simulink model "TP_1"  (R2018a)
settings: Solver=VariableStepAuto  StartTime=0.0  StopTime=500  RelTol=1e-3
settings Model: Creator=akumar2017  LastModifiedBy=Frank NGO

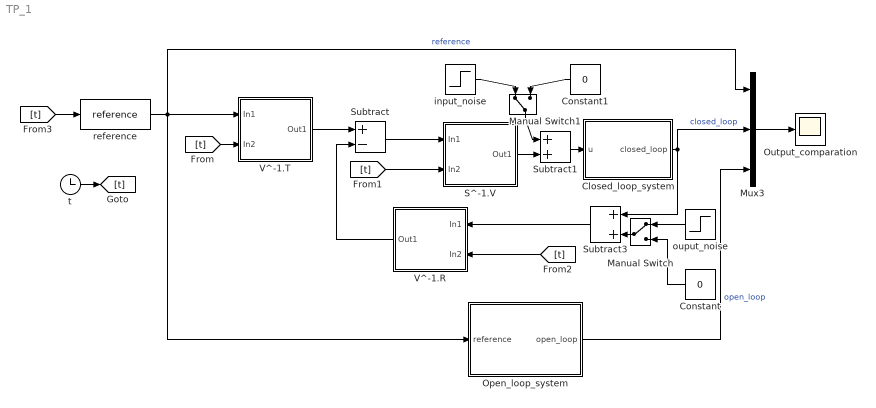
== system TP_1 ==
  Closed_loop_system : Subsystem
  Constant : Constant  Value=0
  Constant1 : Constant  Value=0
  Manual Switch : ManualSwitch
  Manual Switch1 : ManualSwitch
  Mux3 : Mux  Inputs=3
  Open_loop_system : Subsystem
  Output_comparation : Scope
  S^-1.V : Subsystem
  Subtract : Sum  Inputs=+-
  Subtract1 : Sum
  Subtract3 : Sum
  V^-1.R : Subsystem
  V^-1.T : Subsystem
  input_noise : Step  Time=100  After=5  SampleTime=0
  ouput_noise : Step  Time=200  After=0.09  SampleTime=0
  reference : MATLABFcn  MATLABFcn=reference  OutputDimensions=1
  t : Clock
  wires:
  Closed_loop_system/1(closed_loop) -> Subtract3/1, Mux3/2  "closed_loop"
  [t] -> V^-1.T/2(In2)
  [t] -> S^-1.V/2(In2)
  t/1 -> [t]
  [t] -> V^-1.R/2(In2)
  V^-1.T/1(Out1) -> Subtract/1
  V^-1.R/1(Out1) -> Subtract/2
  Subtract/1 -> S^-1.V/1(In1)
  Mux3/1 -> Output_comparation/1
  [t] -> reference/1
  S^-1.V/1(Out1) -> Subtract1/2
  Subtract1/1 -> Closed_loop_system/1(u)
  input_noise/1 -> Manual Switch1/1
  reference/1 -> Open_loop_system/1(reference), Mux3/1, V^-1.T/1(In1)  "reference"
  Subtract3/1 -> V^-1.R/1(In1)
  ouput_noise/1 -> Manual Switch/1
  Open_loop_system/1(open_loop) -> Mux3/3  "open_loop"
  Constant/1 -> Manual Switch/2
  Manual Switch/1 -> Subtract3/2
  Manual Switch1/1 -> Subtract1/1
  Constant1/1 -> Manual Switch1/2

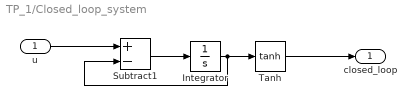
== system TP_1/Closed_loop_system ==
  u : Inport
  Integrator : Integrator
  Subtract1 : Sum  Inputs=+-
  Tanh : Trigonometry  Operator=tanh
  closed_loop : Outport
  wires:
  Subtract1/1 -> Integrator/1
  Integrator/1 -> Subtract1/2, Tanh/1
  Tanh/1 -> closed_loop/1
  u/1 -> Subtract1/1

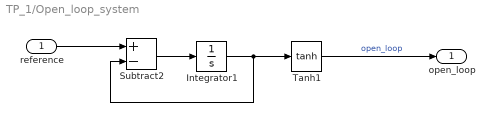
== system TP_1/Open_loop_system ==
  reference : Inport
  Integrator1 : Integrator
  Subtract2 : Sum  Inputs=+-
  Tanh1 : Trigonometry  Operator=tanh
  open_loop : Outport
  wires:
  Integrator1/1 -> Subtract2/2, Tanh1/1
  Subtract2/1 -> Integrator1/1
  reference/1 -> Subtract2/1
  Tanh1/1 -> open_loop/1  "open_loop"

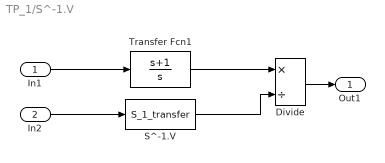
== system TP_1/S^-1.V ==
  In1 : Inport
  In2 : Inport  Port=2
  Divide : Product  Inputs=*/
  S^-1.V : MATLABFcn  MATLABFcn=S_1_transfer  OutputDimensions=1
  Transfer Fcn1 : TransferFcn  Numerator=[1 1]  Denominator=[1 0]
  Out1 : Outport
  wires:
  Transfer Fcn1/1 -> Divide/1
  In1/1 -> Transfer Fcn1/1
  In2/1 -> S^-1.V/1
  Divide/1 -> Out1/1
  S^-1.V/1 -> Divide/2

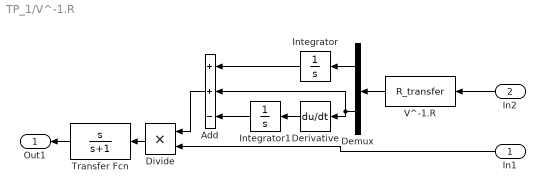
== system TP_1/V^-1.R ==
  In1 : Inport
  In2 : Inport  Port=2
  Add : Sum  Inputs=++-
  Demux : Demux  Outputs=2
  Derivative : Derivative
  Divide : Product  Inputs=**
  Integrator : Integrator
  Integrator1 : Integrator
  Transfer Fcn : TransferFcn  Numerator=[1 0]  Denominator=[1 1]
  V^-1.R : MATLABFcn  MATLABFcn=R_transfer
  Out1 : Outport
  wires:
  In1/1 -> Divide/2
  V^-1.R/1 -> Demux/1
  Integrator/1 -> Add/1
  Add/1 -> Divide/1
  Transfer Fcn/1 -> Out1/1
  Derivative/1 -> Integrator1/1
  Integrator1/1 -> Add/3
  Demux/2 -> Derivative/1, Add/2
  Demux/1 -> Integrator/1
  In2/1 -> V^-1.R/1
  Divide/1 -> Transfer Fcn/1

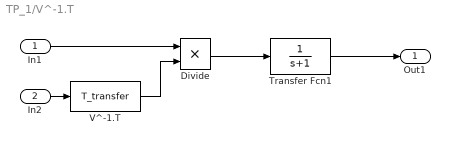
== system TP_1/V^-1.T ==
  In1 : Inport
  In2 : Inport  Port=2
  Divide : Product  Inputs=**
  Transfer Fcn1 : TransferFcn  Denominator=[1 1]
  V^-1.T : MATLABFcn  MATLABFcn=T_transfer  OutputDimensions=1
  Out1 : Outport
  wires:
  In1/1 -> Divide/1
  Transfer Fcn1/1 -> Out1/1
  Divide/1 -> Transfer Fcn1/1
  In2/1 -> V^-1.T/1
  V^-1.T/1 -> Divide/2
